simulink subsystem "rocket_plant"  (R2024b)
settings: Solver=VariableStepAuto  StartTime=0.0  StopTime=10.0  RelTol=1e-3
undefined symbols (not defined in the file or in its folder): location, Mdot, OR_cg, rail_angle, sim_time, time_idle
libraries: shared6dof x1
settings Model: Creator=joedo  LastModifiedBy=finnb

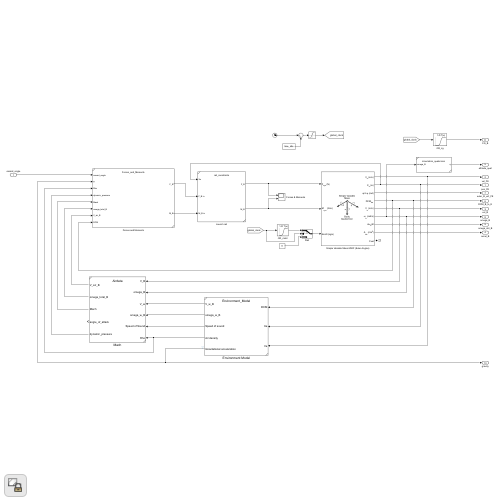
[thumbnail: Simulink's stored preview of the top-level diagram]
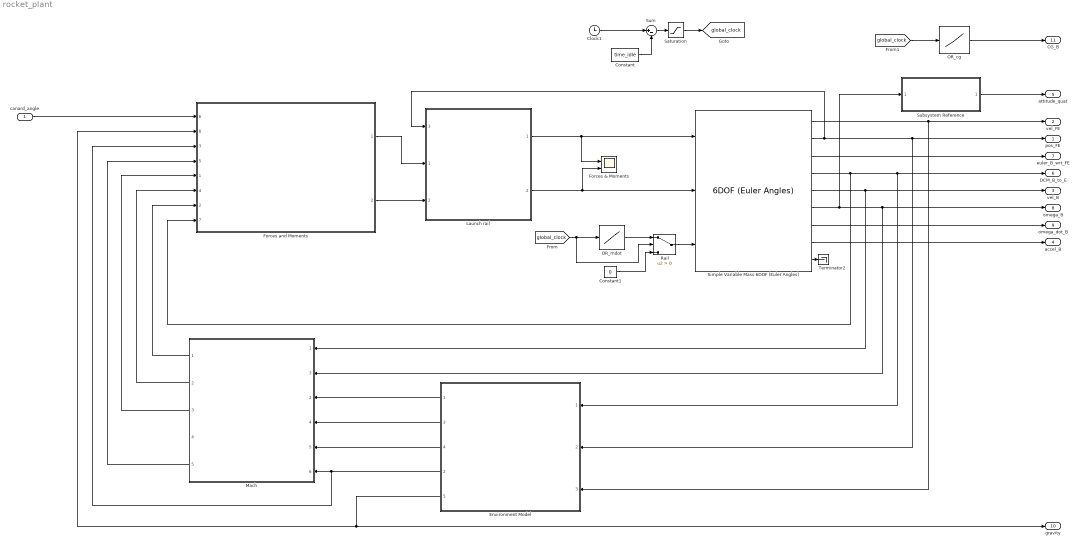
== system rocket_plant ==
  canard_angle : Inport
  Clock1 : Clock
  Constant : Constant  Value=time_idle
  Constant1 : Constant  Value=0
  Environment Model : Subsystem  ReferencedSubsystem=Environment_Model
      settings: PortSchema="{\"entries\":[{\"content\":{\"sides\":[{\"content\":{\"connectorIds\":[\"In1\",\"In2\",\"In3\"]},\"type\":\"ConnectorPlacement.EquallySpacedRectSide\",\"uuid\":\"64123a32-a932-4412-b231-f124dbdf971a\"},{\"content\":{\"connectorIds\":[\"Out1\",\"Out3\",\"Out4\",\"Out2\",\"Out5\"],\"side\":\"RIGHT\"},\"type\":\"ConnectorPlacement.EquallySpacedRectSide\",\"uuid\":\"0f612281-bb96-4498-9d58-547a9e7732cf\"},{\"content\":{\"side\":\"TOP\"},\"type\":\"ConnectorPlacement.EquallySpacedRectSide\",\"uuid\":\"c2030a30-3ec3-4766-b151-459d51387a64\"}]},\"type\":\"ConnectorPlacement.EquallySpacedConnector\",\"uuid\":\"82590f51-359e-4aa6-8371-32bd0e860417\"}],\"packageUris\":[\"http://schema.mathworks.com/mf0/Connector/R2020b\"],\"version\":\"1.0\"}"
  Forces & Moments : Scope  NumInputPorts=2
  "Forces and Moments " : Subsystem  ReferencedSubsystem=Forces_and_Moments
      settings: PortSchema="{\"entries\":[{\"content\":{\"sides\":[{\"content\":{\"connectorIds\":[\"In6\",\"In8\",\"In3\",\"In5\",\"In1\",\"In4\",\"In2\",\"In7\"]},\"type\":\"ConnectorPlacement.EquallySpacedRectSide\",\"uuid\":\"fd13fb59-2e30-4a01-81c3-5431a883c164\"},{\"content\":{\"connectorIds\":[\"Out1\",\"Out2\"],\"side\":\"RIGHT\"},\"type\":\"ConnectorPlacement.EquallySpacedRectSide\",\"uuid\":\"3e8c7c69-66ff-4235-96d1-b8c4a6a79afe\"},{\"content\":{\"side\":\"TOP\"},\"type\":\"ConnectorPlacement.EquallySpacedRectSide\",\"uuid\":\"87d2252f-d21b-4c01-befc-b19bdbbce934\"},{\"content\":{\"side\":\"BOTTOM\"},\"type\":\"ConnectorPlacement.EquallySpacedRectSide\",\"uuid\":\"ec09fd7f-a26c-44e7-8cf9-dc1263f83c25\"}]},\"type\":\"ConnectorPlacement.EquallySpacedConnector\",\"uuid\":\"11501969-d7f2-4657-bb2c-ad94eaf213df\"}],\"packageUris\":[\"http://schema.mathworks.com/mf0/Connector/R2020b\"],\"version\":\"1.0\"}"
  Launch rail : Subsystem  ReferencedSubsystem=rail_constraints
      settings: PortSchema="{\"entries\":[{\"content\":{\"sides\":[{\"content\":{\"connectorIds\":[\"In3\",\"In1\",\"In2\"]},\"type\":\"ConnectorPlacement.EquallySpacedRectSide\",\"uuid\":\"f8bc89cf-4366-4095-a699-e573bc22001a\"},{\"content\":{\"connectorIds\":[\"Out1\",\"Out2\"],\"side\":\"RIGHT\"},\"type\":\"ConnectorPlacement.EquallySpacedRectSide\",\"uuid\":\"f55d6fa0-3d5e-48fa-b07b-9e72276225fb\"},{\"content\":{\"side\":\"TOP\"},\"type\":\"ConnectorPlacement.EquallySpacedRectSide\",\"uuid\":\"5696589c-23a4-46a9-b349-1864b914459a\"}]},\"type\":\"ConnectorPlacement.EquallySpacedConnector\",\"uuid\":\"1b8f695c-cf97-4880-abd1-8dadf97d6ecb\"}],\"packageUris\":[\"http://schema.mathworks.com/mf0/Connector/R2020b\"],\"version\":\"1.0\"}"
  Mach : Subsystem  ReferencedSubsystem=Airdata
      settings: PortSchema="{\"entries\":[{\"content\":{\"sides\":[{\"content\":{\"connectorIds\":[\"In1\",\"In3\",\"In2\",\"In4\",\"In5\",\"In6\"]},\"type\":\"ConnectorPlacement.EquallySpacedRectSide\",\"uuid\":\"db51eaac-c0b2-4518-b505-d133d5b16a6c\"},{\"content\":{\"connectorIds\":[\"Out1\",\"Out2\",\"Out3\",\"Out4\",\"Out5\"],\"side\":\"RIGHT\"},\"type\":\"ConnectorPlacement.EquallySpacedRectSide\",\"uuid\":\"a7fd795c-a715-4c77-8ba1-be4eead1e898\"},{\"content\":{\"side\":\"TOP\"},\"type\":\"ConnectorPlacement.EquallySpacedRectSide\",\"uuid\":\"b6799e08-e3b2-4190-9d60-cc990e08ae9b\"}]},\"type\":\"ConnectorPlacement.EquallySpacedConnector\",\"uuid\":\"c4754658-7600-454e-bcfb-80ce705a6bc7\"}],\"packageUris\":[\"http://schema.mathworks.com/mf0/Connector/R2020b\"],\"version\":\"1.0\"}"
  OR_cg : Lookup_n-D  NumberOfTableDimensions=1  BreakpointsForDimension1=sim_time  Table=OR_cg  InternalRulePriority=Speed  RndMeth=Simplest
  OR_mdot : Lookup_n-D  NumberOfTableDimensions=1  BreakpointsForDimension1=sim_time  Table=Mdot  InternalRulePriority=Speed  RndMeth=Simplest
  Rail : Switch  Criteria=u2 > Threshold  SaturateOnIntegerOverflow=off  InputSameDT=off
  Saturation : Saturate  UpperLimit=inf  LowerLimit=0
  Simple Variable Mass 6DOF (Euler Angles) : shared6dof/6DOF (Euler Angles)  units=Metric (MKS)  mtype=Simple Variable  rep=Quaternion  xme_0=[location(1) 0 0]  Vm_0=[0 0 0]  eul_0=[0 rail_angle 0]  pm_0=[0 0 0]  mass_0=total_mass_0  mass_e=total_mass_d  mass_f=total_mass_0  inertia=eye(3)  inertia_e=I_d  inertia_f=I_0  k_quat=1.0  vre_flag=off  abi_flag=off  aMode=aMode  xme_statename=''  Vm_statename=''  eul_statename=''  quat_statename=''  pm_statename=''  mass_statename=''
  Subsystem Reference : Subsystem  ReferencedSubsystem=kinematics_quaternion
  Sum : Sum  Inputs=|+-
  Terminator2 : Terminator
  pos_FE : Outport
  vel_FE : Outport  Port=2
  vel_B : Outport  Port=3
  accel_B : Outport  Port=4
  attitude_quat : Outport  Port=5
  DCM_B_to_E : Outport  Port=6
  euler_B_wrt_FE : Outport  Port=7
  omega_B : Outport  Port=8
  omega_dot_B : Outport  Port=9
  gravity : Outport  Port=10
  CG_B : Outport  Port=11
  tag scope: global_clock=global
  wires:
  Launch rail/1 -> Forces & Moments/1, Simple Variable Mass 6DOF (Euler Angles)/1
  canard_angle/1 -> "Forces and Moments "/6
  Simple Variable Mass 6DOF (Euler Angles)/6 -> omega_B/1, Mach/3, Subsystem Reference/1
  Simple Variable Mass 6DOF (Euler Angles)/5 -> vel_B/1, Mach/1
  Environment Model/1 -> Mach/2
  Mach/2 -> "Forces and Moments "/4
  Environment Model/3 -> Mach/4
  Environment Model/2 -> "Forces and Moments "/3, Mach/6
  Launch rail/2 -> Forces & Moments/2, Simple Variable Mass 6DOF (Euler Angles)/2
  Environment Model/4 -> Mach/5
  Simple Variable Mass 6DOF (Euler Angles)/2 -> Environment Model/2, pos_FE/1, Launch rail/3
  Mach/3 -> "Forces and Moments "/1
  OR_mdot/1 -> Rail/1
  Simple Variable Mass 6DOF (Euler Angles)/8 -> accel_B/1
  Simple Variable Mass 6DOF (Euler Angles)/9 -> Terminator2/1
  Environment Model/5 -> "Forces and Moments "/8, gravity/1
  Simple Variable Mass 6DOF (Euler Angles)/1 -> Environment Model/3, vel_FE/1
  Simple Variable Mass 6DOF (Euler Angles)/3 -> euler_B_wrt_FE/1
  Simple Variable Mass 6DOF (Euler Angles)/7 -> omega_dot_B/1
  Simple Variable Mass 6DOF (Euler Angles)/4 -> Environment Model/1, DCM_B_to_E/1, "Forces and Moments "/7
  [global_clock] -> Rail/2, OR_mdot/1
  Rail/1 -> Simple Variable Mass 6DOF (Euler Angles)/3
  Constant1/1 -> Rail/3
  [global_clock] -> OR_cg/1
  OR_cg/1 -> CG_B/1
  Clock1/1 -> Sum/1
  Sum/1 -> Saturation/1
  Constant/1 -> Sum/2
  Saturation/1 -> [global_clock]
  Subsystem Reference/1 -> attitude_quat/1
  Mach/1 -> "Forces and Moments "/2
  Mach/5 -> "Forces and Moments "/5
  "Forces and Moments "/1 -> Launch rail/1
  "Forces and Moments "/2 -> Launch rail/2
